simulink model "plc_code_test"  (R2013a)
settings: Solver=FixedStepDiscrete  StartTime=0.0  StopTime=10.0  RelTol=1e-3
settings Model: Creator=Administrator  LastModifiedBy=Administrator
settings DebuggingCC: BusObjectLabelMismatch=error
settings ConfigComp: Description=PLC Coder Custom Configuration Component  PLC_OutputDir=./plcsrc  PLC_TargetIDE=rslogix5000_routine  PLC_GenerateReport=off

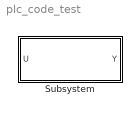
== system plc_code_test ==
  Subsystem : Subsystem  TreatAsAtomicUnit=on

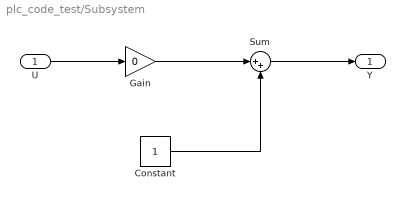
== system plc_code_test/Subsystem ==
  U : Inport
  Constant : Constant
  Gain : Gain  Gain=0
  Sum : Sum  Inputs=|++
  Y : Outport
  wires:
  U/1 -> Gain/1
  Gain/1 -> Sum/1
  Constant/1 -> Sum/2
  Sum/1 -> Y/1
